simulink model "Worked_Example_3_4"  (R2024b)
settings: Solver=VariableStepAuto  StartTime=0.0  StopTime=60  RelTol=1e-3
settings Model: Creator=GH-X-ST  LastModifiedBy=GH-X-ST

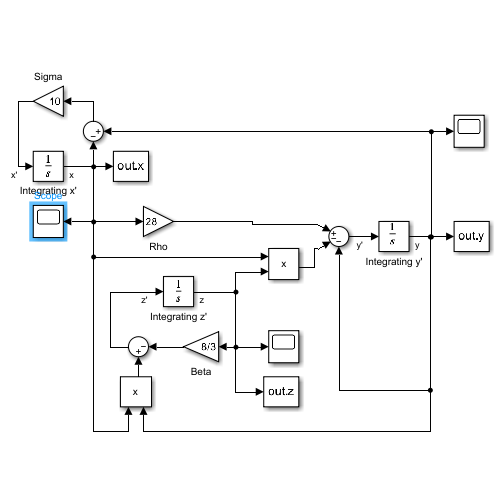
[thumbnail: Simulink's stored preview of the top-level diagram]
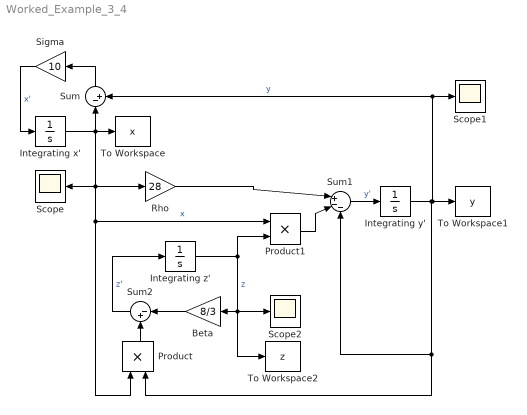
== system Worked_Example_3_4 ==
  Beta : Gain  Gain=8/3
  Integrating x' : Integrator  InitialCondition=-8.1
  Integrating y' : Integrator  InitialCondition=8
  Integrating z' : Integrator  InitialCondition=27
  Product : Product
  Product1 : Product
  Rho : Gain  Gain=28
  Scope : Scope
  Scope1 : Scope
  Scope2 : Scope
  Sigma : Gain  Gain=10
  Sum : Sum  Inputs=|-+
  Sum1 : Sum  Inputs=|+--
  Sum2 : Sum  Inputs=|-+
  To Workspace : ToWorkspace  VariableName=x  SaveFormat=Structure With Time  SampleTime=-1
  To Workspace1 : ToWorkspace  VariableName=y  SaveFormat=Structure With Time  SampleTime=-1
  To Workspace2 : ToWorkspace  VariableName=z  SaveFormat=Structure With Time  SampleTime=-1
  wires:
  Sigma/1 -> Integrating x'/1  "x'"
  Integrating x'/1 -> To Workspace/1, Sum/1, Scope/1, Rho/1, Product/1, Product1/1  "x"
  Sum/1 -> Sigma/1
  Rho/1 -> Sum1/1
  Beta/1 -> Sum2/1
  Integrating y'/1 -> To Workspace1/1, Sum/2, Scope1/1, Sum1/3, Product/2  "y"
  Integrating z'/1 -> Scope2/1, To Workspace2/1, Beta/1, Product1/2  "z"
  Product1/1 -> Sum1/2
  Sum1/1 -> Integrating y'/1  "y'"
  Product/1 -> Sum2/2
  Sum2/1 -> Integrating z'/1  "z'"
